simulink model "lab_10_simulink_comp"  (R2024b)
settings: Solver=ode45  StartTime=0.0  StopTime=150  MaxStep=0.05  RelTol=1e-3
libraries: simulink x2
settings Model: Creator=lw53894  LastModifiedBy=lw53894

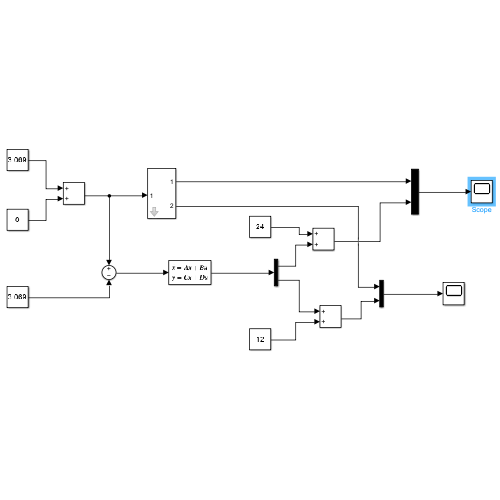
[thumbnail: Simulink's stored preview of the top-level diagram]
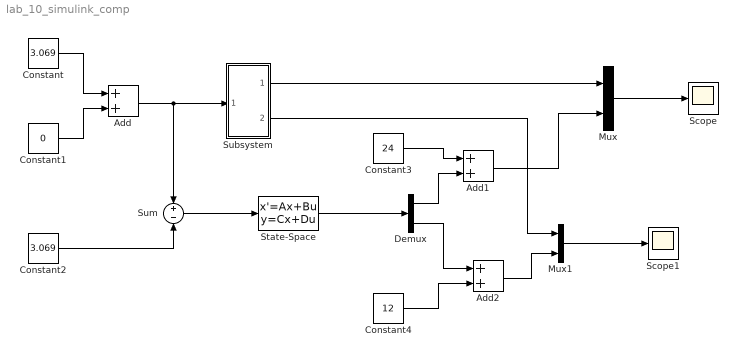
== system lab_10_simulink_comp ==
  Add : Sum
  Add1 : Sum
  Add2 : Sum
  Constant : Constant  Value=3.069
  Constant1 : Constant  Value=0
  Constant2 : Constant  Value=3.069
  Constant3 : Constant  Value=24
  Constant4 : Constant  Value=12
  Demux : Demux  Outputs=2
  Mux : Mux  Inputs=2
  Mux1 : Mux  Inputs=2
  Scope : Scope
  Scope1 : Scope
  State-Space : StateSpace  A=[-0.1279 0.1279; 0.0639 -0.1279]  B=[1;0]  C=[1 0;0 1]  D=[0;0]  InitialCondition=[-20 -10]
  Subsystem : Subsystem  mask{h1=4, h2=2, S1=1, S2=2, Swy1=0.2, Swy2=0.2, fi1=1, fi2=1, g=9.81, Qwe=0}
  Sum : Sum  Inputs=+-
  wires:
  Add/1 -> Sum/1, Subsystem/1(In1)
  Constant1/1 -> Add/2
  Constant/1 -> Add/1
  Constant2/1 -> Sum/2
  Sum/1 -> State-Space/1
  Subsystem/1(Out1) -> Mux/1
  State-Space/1 -> Demux/1
  Constant3/1 -> Add1/1
  Demux/1 -> Add1/2
  Add1/1 -> Mux/2
  Mux/1 -> Scope/1
  Constant4/1 -> Add2/2
  Demux/2 -> Add2/1
  Add2/1 -> Mux1/2
  Subsystem/2(Out2) -> Mux1/1
  Mux1/1 -> Scope1/1

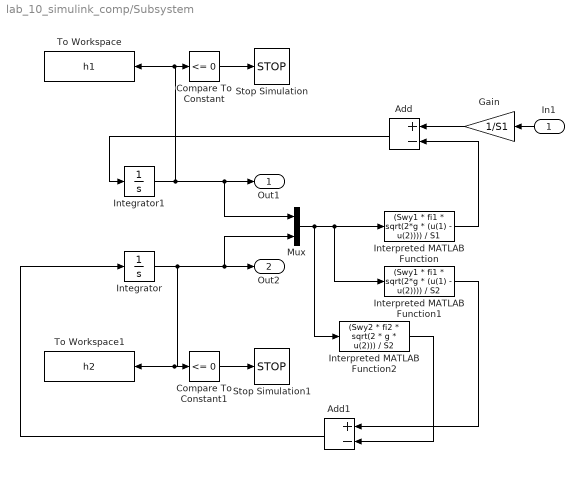
== system lab_10_simulink_comp/Subsystem ==
  In1 : Inport
  Add : Sum  Inputs=+-
  Add1 : Sum  Inputs=+-
  Compare To Constant : simulink/Logic and Bit Operations/Compare To Constant  relop=<=  const=0  OutDataTypeStr=boolean
  Compare To Constant1 : simulink/Logic and Bit Operations/Compare To Constant  relop=<=  const=0  OutDataTypeStr=boolean
  Gain : Gain  Gain=1/S1
  Integrator : Integrator  InitialCondition=h2
  Integrator1 : Integrator  InitialCondition=h1
  Interpreted MATLAB Function : MATLABFcn  MATLABFcn=(Swy1 * fi1 * sqrt(2*g * (u(1) - u(2)))) / S1
  Interpreted MATLAB Function1 : MATLABFcn  MATLABFcn=(Swy1 * fi1 * sqrt(2*g * (u(1) - u(2)))) / S2
  Interpreted MATLAB Function2 : MATLABFcn  MATLABFcn=(Swy2 * fi2 * sqrt(2 * g * u(2))) / S2
  Mux : Mux  Inputs=2
  Stop Simulation : Stop
  Stop Simulation1 : Stop
  To Workspace : ToWorkspace  VariableName=h1  SaveFormat=Timeseries  SampleTime=-1
  To Workspace1 : ToWorkspace  VariableName=h2  SaveFormat=Timeseries  SampleTime=-1
  Out1 : Outport
  Out2 : Outport  Port=2
  wires:
  Mux/1 -> Interpreted MATLAB Function2/1, Interpreted MATLAB Function1/1, Interpreted MATLAB Function/1
  Integrator1/1 -> To Workspace/1, Compare To Constant/1, Out1/1, Mux/1
  Integrator/1 -> To Workspace1/1, Compare To Constant1/1, Out2/1, Mux/2
  Compare To Constant/1 -> Stop Simulation/1
  Compare To Constant1/1 -> Stop Simulation1/1
  In1/1 -> Gain/1
  Add/1 -> Integrator1/1
  Interpreted MATLAB Function/1 -> Add/2
  Gain/1 -> Add/1
  Interpreted MATLAB Function1/1 -> Add1/1
  Interpreted MATLAB Function2/1 -> Add1/2
  Add1/1 -> Integrator/1
